simulink model "EPS_theta1input_simpletorquemap_simpletiremodel"  (R2022b)
settings: Solver=ode3  StartTime=0.0  StopTime=15  FixedStep=0.001  RelTol=1e-4  EnableMultiTasking=on
values from neighbouring files (symbols this model uses):
  amp_input_theta1 = amp_input_theta1_deg*pi/180    (= 1.0471975512)    [simulBack_theta1_simple.m]
  assist = 9.3    [simulBack_theta1_simple.m]
  C1 = 0.23    [simulBack_theta1_simple.m]
  C2 = 2.4    [simulBack_theta1_simple.m]
  Carspeed = 100    [simulBack_theta1_simple.m]
  deadband = 0    [simulBack_theta1_simple.m]
  freq_input_theta1 = 10    [simulBack_theta1_simple.m]
  friction_level = 0    [simulBack_theta1_simple.m]
  J1 = 0.033    [simulBack_theta1_simple.m]
  J2 = 0.085    [simulBack_theta1_simple.m]
  K = 143.24    [simulBack_theta1_simple.m]
  lagpole = 50    [simulBack_theta1_simple.m]
  lagzero = 15    [simulBack_theta1_simple.m]
  leadpole = 100    [simulBack_theta1_simple.m]
  leadzero = 10    [simulBack_theta1_simple.m]
  motor_onoff = 1    [simulBack_theta1_simple.m]
  motorcutoff = 100*2*3.14    (= 628)    [simulBack_theta1_simple.m]
  motordelay_onoff = 0    [simulBack_theta1_simple.m]
  noise_var = 0    [simulBack_theta1_simple.m]
  offset_input_theta1 = 0    [simulBack_theta1_simple.m]
  SAT_coefficient = 20/180*pi    (= 0.349065850399)    [simulBack_theta1_simple.m]
  tire_stiffness = 0.51    [simulBack_theta1_simple.m]
  tireangle_max = 60    [simulBack_theta1_simple.m]
settings Model: Creator=Dongwook Lee  LastModifiedBy=LDW
settings SolverCC: AlgebraicLoopSolver=TrustRegion
settings DataIOCC: LimitDataPoints=on  SaveFormat=Array  SignalLoggingSaveFormat=ModelDataLogs  ReturnWorkspaceOutputs=off
settings OptimizationCC: ExpressionDepthLimit=2147483647  LifeSpan=inf
settings DebuggingCC: UnderspecifiedInitializationDetection=Classic  MergeDetectMultiDrivingBlocksExec=none  SolverPrmCheckMsg=warning  FcnCallInpInsideContextMsg=warning  UnconnectedInputMsg=warning  UnconnectedOutputMsg=warning  UnconnectedLineMsg=warning  StateNameClashWarn=warning  SFUnexpectedBacktrackingDiag=warning  SFNoUnconditionalDefaultTransitionDiag=warning  SFExecutionAtInitializationDiag=none  SFMachineParentedDataDiag=warning  ArithmeticOperatorsInVariantConditions=warning
settings HardwareCC: ProdBitPerPointer=32  ProdBitPerSizeT=32  ProdBitPerPtrDiffT=32  ProdLargestAtomicFloat=None  ProdIntDivRoundTo=Undefined  ProdEndianess=Unspecified  ProdWordSize=32  ProdHWDeviceType=32-bit Generic
settings ModelReferenceCC: PropagateSignalLabelsOutOfModel=off
settings SFSimCC: SimUseLocalCustomCode=off  CustomCodeUndefinedFunction=UseInterfaceOnly
settings RTWCC: RTWUseLocalCustomCode=off
settings CodeAppCC: StateflowObjectComments=on
settings GRTTargetCC: TargetLangStandard=C89/C90 (ANSI)  CombineOutputUpdateFcns=off  GRTInterface=on
settings ConfigComp: CovMetricSettings=dw  CovSaveCumulativeToWorkspaceVar=on  CovSaveSingleToWorkspaceVar=on  CovExternalEMLEnable=off  CovSFcnEnable=off

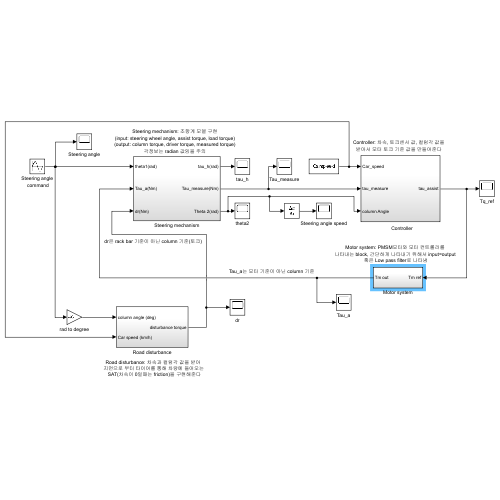
[thumbnail: Simulink's stored preview of the top-level diagram]
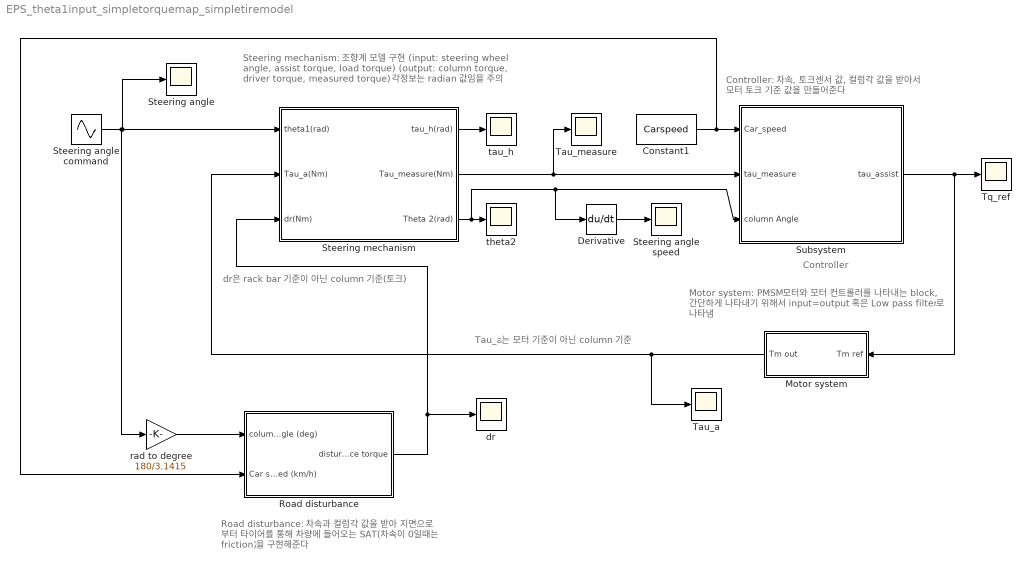
== system EPS_theta1input_simpletorquemap_simpletiremodel ==
  note: dr은 rack bar 기준이 아닌 column 기준(토크)
  note: Tau_a는 모터 기준이 아닌 column 기준
  note: Road disturbance: 차속과 컬럼각 값을 받아
      | 지면으로 부터 타이어를 통해 차량에 들어오는
      |  SAT(차속이 0일때는 friction)을 구현해준다
  note: Motor system: PMSM모터와 모터 컨트롤러를
      | 나타내는 block, 간단하게 나타내기 위해서 input=output
      | 혹은 Low pass filter로 나타냄
  note: Controller: 차속, 토크센서 값, 컬럼각 값을
      | 받아서 모터 토크 기준 값을 만들어준다
  note: Steering mechanism: 조향계 모델 구현
      | (input: steering wheel angle, assist torque, load torque)
      | (output: column torque, driver torque, measured torque)
      | 각정보는 radian 값임을 주의
  note: Controller
  Constant1 : Constant  Value=Carspeed
  Derivative : Derivative
  Motor system : Subsystem
  Road disturbance : Subsystem
  Steering angle : Scope
  Steering angle command : Sin  Amplitude=amp_input_theta1  Bias=offset_input_theta1  Frequency=freq_input_theta1  SampleTime=0
  Steering angle speed : Scope
  Steering mechanism : Subsystem
  Subsystem : Subsystem
  Tau_a : Scope
  Tau_measure : Scope
  Tq_ref : Scope
  dr : Scope
  rad to degree : Gain  Gain=180/3.1415
  tau_h : Scope
  theta2 : Scope
  wires:
  Steering mechanism/1(tau_h(rad)) -> tau_h/1
  Subsystem/1(tau_assist) -> Motor system/1(Tm ref), Tq_ref/1
  Steering mechanism/2(Tau_measure(Nm)) -> Tau_measure/1, Subsystem/2(tau_measure)
  Derivative/1 -> Steering angle speed/1
  Steering mechanism/3(Theta 2(rad)) -> Subsystem/3(column Angle), Derivative/1, theta2/1
  Steering angle command/1 -> Steering angle/1, Steering mechanism/1(theta1(rad)), rad to degree/1
  Constant1/1 -> Road disturbance/2(Car speed (km/h)), Subsystem/1(Car_speed)
  Motor system/1(Tm out) -> Tau_a/1, Steering mechanism/2(Tau_a(Nm))
  rad to degree/1 -> Road disturbance/1(column angle (deg))
  Road disturbance/1(disturbance torque) -> Steering mechanism/3(dr(Nm)), dr/1

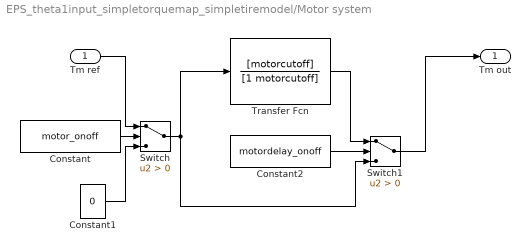
== system EPS_theta1input_simpletorquemap_simpletiremodel/Motor system ==
  Tm ref : Inport
  Constant : Constant  Value=motor_onoff
  Constant1 : Constant  Value=0
  Constant2 : Constant  Value=motordelay_onoff
  Switch : Switch  Criteria=u2 > Threshold  SaturateOnIntegerOverflow=off  InputSameDT=off
  Switch1 : Switch  Criteria=u2 > Threshold  SaturateOnIntegerOverflow=off  InputSameDT=off
  Transfer Fcn : TransferFcn  Numerator=[motorcutoff]  Denominator=[1 motorcutoff]
  Tm out : Outport
  wires:
  Constant/1 -> Switch/2
  Tm ref/1 -> Switch/1
  Constant1/1 -> Switch/3
  Constant2/1 -> Switch1/2
  Switch1/1 -> Tm out/1
  Switch/1 -> Transfer Fcn/1, Switch1/3
  Transfer Fcn/1 -> Switch1/1

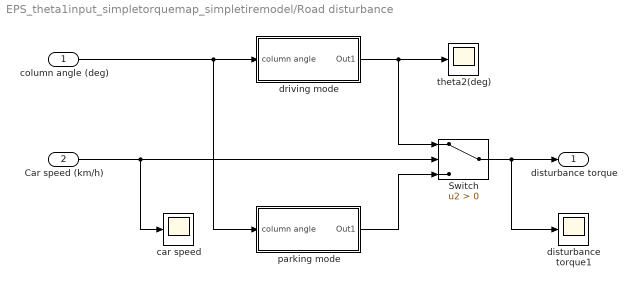
== system EPS_theta1input_simpletorquemap_simpletiremodel/Road disturbance ==
  column angle (deg) : Inport
  Car speed (km/h) : Inport  Port=2
  Switch : Switch  Criteria=u2 > Threshold  SaturateOnIntegerOverflow=off  InputSameDT=off
  car speed : Scope
  disturbance torque1 : Scope
  driving mode : Subsystem
  parking mode : Subsystem
  theta2(deg) : Scope
  disturbance torque : Outport
  wires:
  column angle (deg)/1 -> parking mode/1(column angle), driving mode/1(column angle)
  Car speed (km/h)/1 -> car speed/1, Switch/2
  driving mode/1(Out1) -> theta2(deg)/1, Switch/1
  parking mode/1(Out1) -> Switch/3
  Switch/1 -> disturbance torque/1, disturbance torque1/1

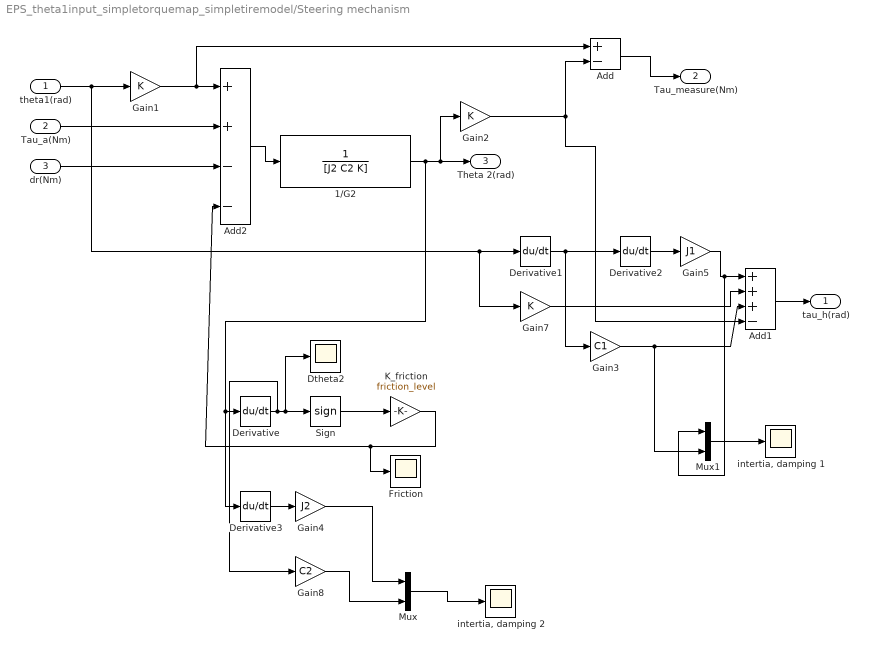
== system EPS_theta1input_simpletorquemap_simpletiremodel/Steering mechanism ==
  theta1(rad) : Inport
  Tau_a(Nm) : Inport  Port=2
  dr(Nm) : Inport  Port=3
  1/G2 : TransferFcn  Denominator=[J2 C2 K]
  Add : Sum  Inputs=+-
  Add1 : Sum  Inputs=+++-
  Add2 : Sum  Inputs=++--
  Derivative{,1..3} (4 alike) : Derivative
  Dtheta2 : Scope
  Friction : Scope
  Gain1 : Gain  Gain=K
  Gain2 : Gain  Gain=K
  Gain3 : Gain  Gain=C1
  Gain4 : Gain  Gain=J2
  Gain5 : Gain  Gain=J1
  Gain7 : Gain  Gain=K
  Gain8 : Gain  Gain=C2
  K_friction : Gain  Gain=friction_level
  Mux : Mux  Inputs=2
  Mux1 : Mux  Inputs=2
  Sign : Signum
  "intertia, damping 1" : Scope
  "intertia, damping 2" : Scope
  tau_h(rad) : Outport
  Tau_measure(Nm) : Outport  Port=2
  Theta 2(rad) : Outport  Port=3
  wires:
  theta1(rad)/1 -> Derivative1/1, Gain7/1, Gain1/1
  Gain1/1 -> Add/1, Add2/1
  Tau_a(Nm)/1 -> Add2/2
  Add2/1 -> 1/G2/1
  1/G2/1 -> Derivative3/1, Derivative/1, Theta 2(rad)/1, Gain2/1
  Gain2/1 -> Add/2, Add1/4
  Derivative/1 -> Gain8/1, Sign/1, Dtheta2/1
  Sign/1 -> K_friction/1
  K_friction/1 -> Add2/4, Friction/1
  Add/1 -> Tau_measure(Nm)/1
  dr(Nm)/1 -> Add2/3
  Derivative1/1 -> Derivative2/1, Gain3/1
  Derivative2/1 -> Gain5/1
  Gain5/1 -> Mux1/1, Add1/1
  Gain3/1 -> Mux1/2, Add1/3
  Add1/1 -> tau_h(rad)/1
  Gain7/1 -> Add1/2
  Mux1/1 -> "intertia, damping 1"/1
  Derivative3/1 -> Gain4/1
  Gain4/1 -> Mux/1
  Gain8/1 -> Mux/2
  Mux/1 -> "intertia, damping 2"/1

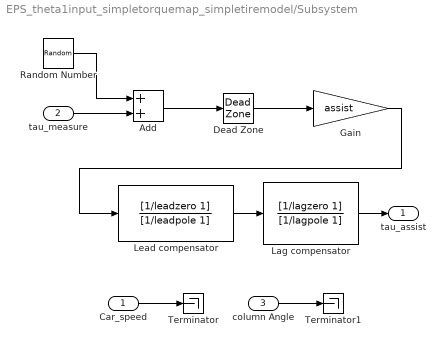
== system EPS_theta1input_simpletorquemap_simpletiremodel/Subsystem ==
  Car_speed : Inport
  tau_measure : Inport  Port=2
  column Angle : Inport  Port=3
  Add : Sum
  Dead Zone : DeadZone  LowerValue=-deadband  UpperValue=deadband
  Gain : Gain  Gain=assist
  Lag compensator : TransferFcn  Numerator=[1/lagzero 1]  Denominator=[1/lagpole 1]
  Lead compensator : TransferFcn  Numerator=[1/leadzero 1]  Denominator=[1/leadpole 1]
  Random Number : RandomNumber  Variance=noise_var  SampleTime=0.001
  Terminator : Terminator
  Terminator1 : Terminator
  tau_assist : Outport
  wires:
  Lead compensator/1 -> Lag compensator/1
  Gain/1 -> Lead compensator/1
  Lag compensator/1 -> tau_assist/1
  Car_speed/1 -> Terminator/1
  column Angle/1 -> Terminator1/1
  tau_measure/1 -> Add/2
  Random Number/1 -> Add/1
  Add/1 -> Dead Zone/1
  Dead Zone/1 -> Gain/1

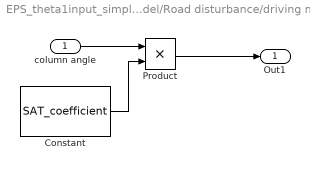
== system EPS_theta1input_simpletorquemap_simpletiremodel/Road disturbance/driving mode ==
  column angle : Inport
  Constant : Constant  Value=SAT_coefficient
  Product : Product
  Out1 : Outport
  wires:
  column angle/1 -> Product/1
  Product/1 -> Out1/1
  Constant/1 -> Product/2

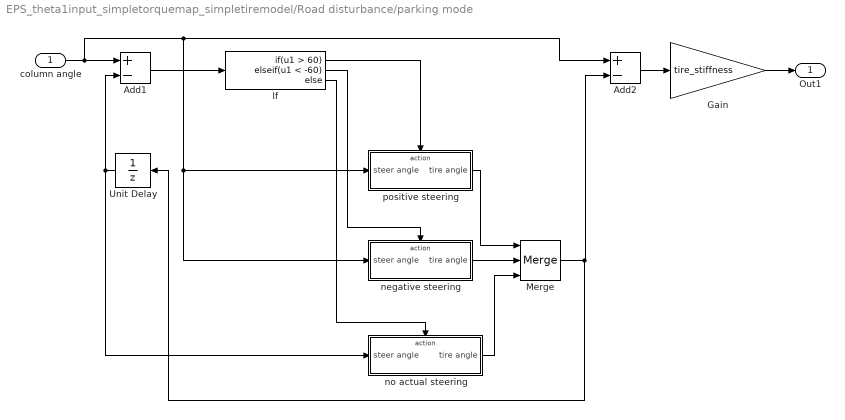
== system EPS_theta1input_simpletorquemap_simpletiremodel/Road disturbance/parking mode ==
  column angle : Inport
  Add1 : Sum  Inputs=+-
  Add2 : Sum  Inputs=+-
  Gain : Gain  Gain=tire_stiffness
  If : If  IfExpression=u1 > 60  ElseIfExpressions=u1 < -60
  Merge : Merge  Inputs=3
  Unit Delay : UnitDelay  SampleTime=-1  HasFrameUpgradeWarning=on
  negative steering : Subsystem  TreatAsAtomicUnit=on
  no actual steering : Subsystem  TreatAsAtomicUnit=on
  positive steering : Subsystem  TreatAsAtomicUnit=on
  Out1 : Outport
  wires:
  column angle/1 -> positive steering/1(steer angle), negative steering/1(steer angle), Add2/1, Add1/1
  Add1/1 -> If/1
  If/1 -> positive steering/Action
  If/2 -> negative steering/Action
  If/3 -> no actual steering/Action
  Unit Delay/1 -> Add1/2, no actual steering/1(steer angle)
  positive steering/1(tire angle) -> Merge/1
  negative steering/1(tire angle) -> Merge/2
  no actual steering/1(tire angle) -> Merge/3
  Merge/1 -> Unit Delay/1, Add2/2
  Add2/1 -> Gain/1
  Gain/1 -> Out1/1

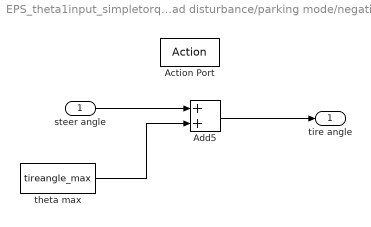
== system EPS_theta1input_simpletorquemap_simpletiremodel/Road disturbance/parking mode/negative steering ==
  steer angle : Inport
  Action Port : ActionPort  ActionPortLabel=elseif { }
  Add5 : Sum
  theta max : Constant  Value=tireangle_max
  tire angle : Outport
  wires:
  steer angle/1 -> Add5/1
  theta max/1 -> Add5/2
  Add5/1 -> tire angle/1

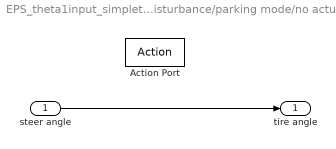
== system EPS_theta1input_simpletorquemap_simpletiremodel/Road disturbance/parking mode/no actual steering ==
  steer angle : Inport
  Action Port : ActionPort  ActionPortLabel=else { }
  tire angle : Outport
  wires:
  steer angle/1 -> tire angle/1

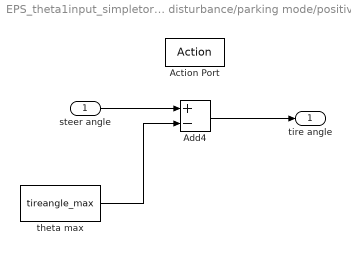
== system EPS_theta1input_simpletorquemap_simpletiremodel/Road disturbance/parking mode/positive steering ==
  steer angle : Inport
  Action Port : ActionPort  ActionPortLabel=if { }
  Add4 : Sum  Inputs=+-
  theta max : Constant  Value=tireangle_max
  tire angle : Outport
  wires:
  steer angle/1 -> Add4/1
  theta max/1 -> Add4/2
  Add4/1 -> tire angle/1
